simulink model "bias_estimate_Franklin"  (R2023a)
settings: Solver=VariableStepAuto  StartTime=0.0  StopTime=50  RelTol=1e-3
values from neighbouring files (symbols this model uses):
  Ad = sysd_plant.A    [bias_param.m]
  Bd = sysd_plant.B    [bias_param.m]
  Cd = sysd_plant.C    [bias_param.m]
  Dd = sysd_plant.D    [bias_param.m]
  Lp = place(Aob',Cob',P)'    [bias_param.m]
  Nx = [1.0;0]    [bias_param.m]
  ref = 10.0    (= 10)    [bias_param.m]
  Ts = 0.10    (= 0.1)    [bias_param.m]
undefined symbols (not defined in the file or in its folder): Kgain
settings Model: Creator=Admin  LastModifiedBy=Admin
settings ModelReferenceCC: EnableRefExpFcnMdlSchedulingChecks=on

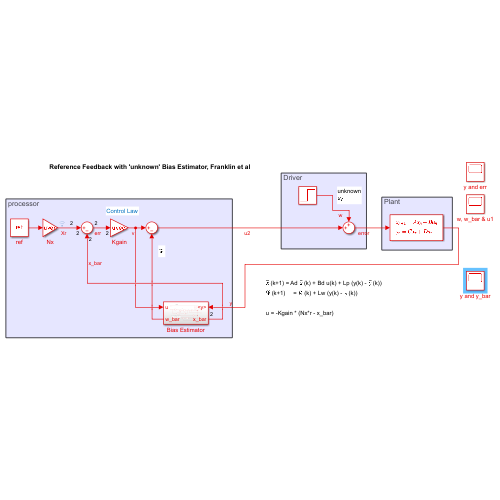
[thumbnail: Simulink's stored preview of the top-level diagram]
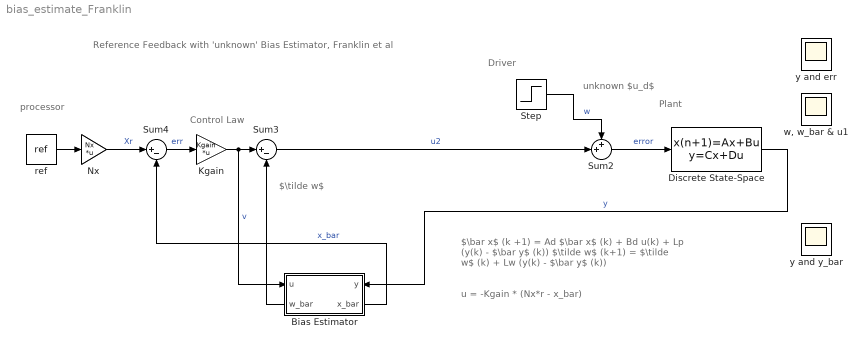
== system bias_estimate_Franklin ==
  note: Driver
  note: processor
  note: u = -Kgain * (Nx*r - x_bar)
  note: Control Law
  note: Plant
  note: Reference Feedback with 'unknown' Bias Estimator, Franklin et al
  note: unknown
      | $u_d$
  note: $\tilde w$
  note: $\bar x$ (k +1) = Ad $\bar x$ (k) + Bd u(k) + Lp (y(k) - $\bar y$ (k))
      | $\tilde w$ (k+1) = $\tilde w$ (k) + Lw (y(k) - $\bar y$ (k))
  Bias Estimator : Subsystem
      settings: PortSchema="{\"entries\":[{\"content\":{\"sides\":[{\"content\":{\"connectorIds\":[\"In1\",\"Out2\"]},\"type\":\"ConnectorPlacement.EquallySpacedRectSide\",\"uuid\":\"f8343b5f-cced-4eae-9acf-824a3500992e\"},{\"content\":{\"connectorIds\":[\"In2\",\"Out1\"],\"side\":\"RIGHT\"},\"type\":\"ConnectorPlacement.EquallySpacedRectSide\",\"uuid\":\"3b121aac-19d6-4d13-9538-8a3da9d8cbfd\"},{\"content\":{\"side\":\"TOP\"},\"type\":\"ConnectorPlacement.EquallySpacedRectSide\",\"uuid\":\"c4a71e11-7286-45ec-b6c4-c2f025e21920\"}]},\"type\":\"ConnectorPlacement.EquallySpacedConnector\",\"uuid\":\"8e54802e-58f8-4bdf-b572-41c99fefdf0e\"}],\"packageUris\":[\"http://schema.mathworks.com/mf0/Connector/R2020b\"],\"version\":\"1.0\"}"
  Discrete State-Space : DiscreteStateSpace  A=Ad  B=Bd  C=Cd  D=Dd  SampleTime=Ts  StateName=plant
  Kgain : Gain  Gain=Kgain  Multiplication=Matrix(K*u) (u vector)
  Nx : Gain  Gain=Nx  Multiplication=Matrix(K*u) (u vector)
  Step : Step  Time=20  After=2  SampleTime=Ts
  Sum2 : Sum  Inputs=++|
  Sum3 : Sum  Inputs=|+-
  Sum4 : Sum  Inputs=|+-
  ref : Constant  Value=ref  SampleTime=Ts
  "w, w_bar & u1" : Scope
      settings: Floating=on
  y and err : Scope
      settings: Floating=on
  y and y_bar : Scope
      settings: Floating=on
  wires:
  Nx/1 -> Sum4/1  "Xr"
  ref/1 -> Nx/1
  Sum4/1 -> Kgain/1  "err"
  Bias Estimator/1(x_bar) -> Sum4/2  "x_bar"
  Sum2/1 -> Discrete State-Space/1  "error"
  Step/1 -> Sum2/1  "w"
  Discrete State-Space/1 -> Bias Estimator/2(y)  "y"
  Kgain/1 -> Bias Estimator/1(u), Sum3/1  "v"
  Sum3/1 -> Sum2/2  "u2"
  Bias Estimator/2(w_bar) -> Sum3/2

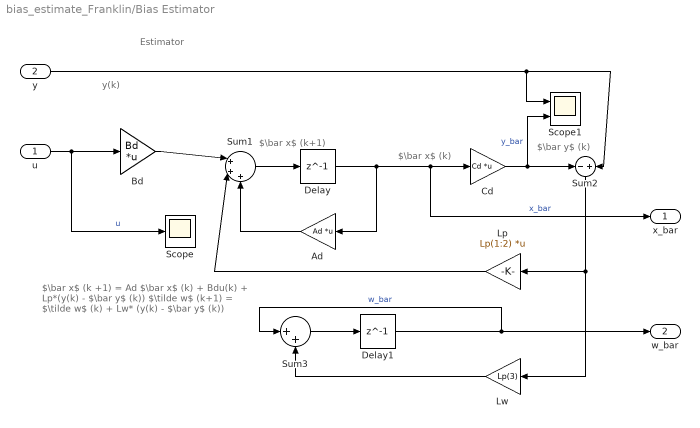
== system bias_estimate_Franklin/Bias Estimator ==
  note: Estimator
  note: $\bar x$ (k)
  note: $\bar x$ (k+1)
  note: $\bar x$ (k +1) = Ad $\bar x$ (k) + Bdu(k) + Lp*(y(k) - $\bar y$ (k))
      | $\tilde w$ (k+1) = $\tilde w$ (k) + Lw* (y(k) - $\bar y$ (k))
  note: y(k)
  note: $\bar y$ (k)
  u : Inport
  y : Inport  Port=2
  Ad : Gain  Gain=Ad  Multiplication=Matrix(K*u) (u vector)
  Bd : Gain  Gain=Bd  Multiplication=Matrix(K*u) (u vector)
  Cd : Gain  Gain=Cd  Multiplication=Matrix(K*u) (u vector)
  Delay : Delay  DelayLength=1  SampleTime=Ts
  Delay1 : Delay  DelayLength=1  SampleTime=Ts
  Lp : Gain  Gain=Lp(1:2)  Multiplication=Matrix(K*u) (u vector)
  Lw : Gain  Gain=Lp(3)
  Scope : Scope
  Scope1 : Scope  NumInputPorts=2
  Sum1 : Sum  Inputs=|+++
  Sum2 : Sum  Inputs=-|+
  Sum3 : Sum  Inputs=|++
  x_bar : Outport
  w_bar : Outport  Port=2
  wires:
  u/1 -> Scope/1, Bd/1  "u"
  Sum1/1 -> Delay/1
  Delay/1 -> Ad/1, x_bar/1, Cd/1  "x_bar"
  Cd/1 -> Scope1/2, Sum2/1  "y_bar"
  y/1 -> Scope1/1, Sum2/2
  Sum2/1 -> Lw/1, Lp/1
  Bd/1 -> Sum1/1
  Ad/1 -> Sum1/3
  Lp/1 -> Sum1/2
  Sum3/1 -> Delay1/1
  Lw/1 -> Sum3/2
  Delay1/1 -> Sum3/1, w_bar/1  "w_bar"
